simulink model "VCUHVACT"  (R2024b)
settings: Solver=FixedStepDiscrete  StartTime=0.0  StopTime=10.0  FixedStep=0.1  RelTol=1e-3
libraries: simulink x10
settings Model: Creator=32032  LastModifiedBy=32032
settings DataIOCC: SaveFormat=StructureWithTime
settings OptimizationCC: DefaultParameterBehavior=Inlined  UseDivisionForNetSlopeComputation=on  InlineInvariantSignals=on  EnhancedBackFolding=on  PassReuseOutputArgsAs=Individual arguments  ZeroExternalMemoryAtStartup=off  ZeroInternalMemoryAtStartup=off  EfficientFloat2IntCast=on  LifeSpan=inf  OptimizeBlockOrder=speed  DifferentSizesBufferReuse=on  EfficientTunableParamExpr=on
settings DebuggingCC: SignalInfNanChecking=error  ParameterTunabilityLossMsg=error  AssertControl=DisableAll  StrictBusMsg=ErrorOnBusTreatedAsVector
settings ModelReferenceCC: ModelReferenceNumInstancesAllowed=Single
settings SFSimCC: CompileTimeRecursionLimit=0  EnableRuntimeRecursion=off  MATLABDynamicMemAlloc=off
settings RTWCC: Description=AUTOSAR  SystemTargetFile=autosar.tlc  GenCodeOnly=on  TemplateMakefile=ert_default_tmf  DataTypeReplacement=CDataTypesFixedWidth
settings CodeAppCC: ForceParamTrailComments=on  IgnoreCustomStorageClasses=off  IgnoreTestpoints=on  OperatorAnnotations=on  SimulinkDataObjDesc=on  SFDataObjDesc=on  MATLABFcnDesc=on  InsertBlockDesc=on
settings STFCustomTargetCC: TargetLangStandard=C99 (ISO)  UtilityFuncGeneration=Shared location  MultiwordLength=256  ParMdlRefBuildCompliant=on  CompOptLevelCompliant=on  IncludeMdlTerminateFcn=off  CombineOutputUpdateFcns=on  SuppressErrorStatus=on  ERTCustomFileBanners=on  SupportAbsoluteTime=off  SupportNonFinite=off  SupportComplex=off  SupportContinuousTime=off  SupportNonInlinedSFcns=off  RemoveResetFunc=on  ParenthesesLevel=Standards  CastingMode=Standards  MATLABClassNameForMDSCustomization=Simulink.SoftwareTarget.ERTCustomization  AutosarCompliant=on  UseToolchainInfoCompliant=on  GenerateSharedConstants=off  LookupTableObjectStructAxisOrder=2,1,3,4,...  LUTObjectStructOrderEvenSpacing=Size,Table,Breakpoints  SystemTargetFile=autosar.tlc
settings ERTTargetCC: TargetLangStandard=C99 (ISO)  UtilityFuncGeneration=Shared location  ConcurrentExecutionCompliant=off  IncludeMdlTerminateFcn=off  SuppressErrorStatus=on  SupportAbsoluteTime=off  SupportNonFinite=off  SupportComplex=off  ParenthesesLevel=Standards  CastingMode=Standards  ModelStepFunctionPrototypeControlCompliant=off  CPPClassGenCompliant=off  AutosarCompliant=on  GenerateSharedConstants=off  LookupTableObjectStructAxisOrder=2,1,3,4,...  LUTObjectStructOrderEvenSpacing=Size,Table,Breakpoints  ERTCustomFileTemplate=example_file_process.tlc  SuppressUnreachableDefaultCases=off  EnableSignedLeftShifts=off  EnableSignedRightShifts=off  BooleanTrueId=TRUE  BooleanFalseId=FALSE
settings ConfigComp: CovScope=ReferencedModels

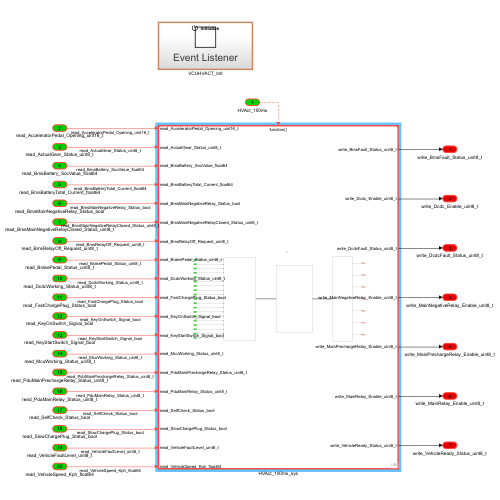
[thumbnail: Simulink's stored preview of the top-level diagram]
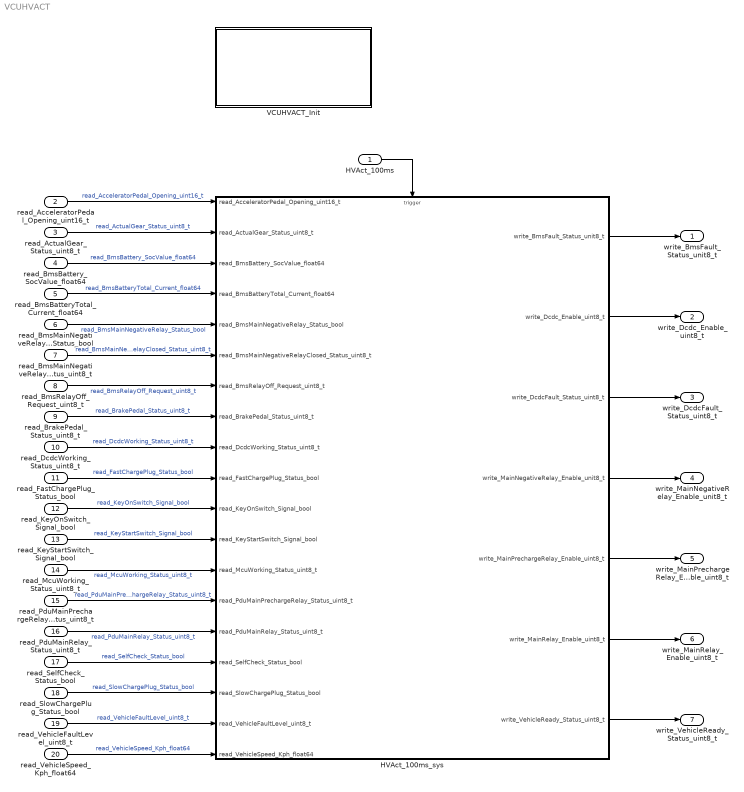
== system VCUHVACT ==
  HVAct_100ms : Inport  SampleTime=0.1  OutputFunctionCall=on
  read_AcceleratorPedal_Opening_uint16_t : Inport  Port=2  OutDataTypeStr=uint16  PortDimensions=1
  read_ActualGear_Status_uint8_t : Inport  Port=3  OutDataTypeStr=uint8  PortDimensions=1
  read_BmsBattery_SocValue_float64 : Inport  Port=4  OutDataTypeStr=double  PortDimensions=1
  read_BmsBatteryTotal_Current_float64 : Inport  Port=5  OutDataTypeStr=double  PortDimensions=1
  read_BmsMainNegativeRelay_Status_bool : Inport  Port=6  OutDataTypeStr=boolean  PortDimensions=1
  read_BmsMainNegativeRelayClosed_Status_uint8_t : Inport  Port=7  OutDataTypeStr=uint8  PortDimensions=1
  read_BmsRelayOff_Request_uint8_t : Inport  Port=8  OutDataTypeStr=uint8  PortDimensions=1
  read_BrakePedal_Status_uint8_t : Inport  Port=9  OutDataTypeStr=uint8  PortDimensions=1
  read_DcdcWorking_Status_uint8_t : Inport  Port=10  OutDataTypeStr=uint8  PortDimensions=1
  read_FastChargePlug_Status_bool : Inport  Port=11  OutDataTypeStr=boolean  PortDimensions=1
  read_KeyOnSwitch_Signal_bool : Inport  Port=12  OutDataTypeStr=boolean  PortDimensions=1
  read_KeyStartSwitch_Signal_bool : Inport  Port=13  OutDataTypeStr=boolean  PortDimensions=1
  read_McuWorking_Status_uint8_t : Inport  Port=14  OutDataTypeStr=uint8  PortDimensions=1
  read_PduMainPrechargeRelay_Status_uint8_t : Inport  Port=15  OutDataTypeStr=uint8  PortDimensions=1
  read_PduMainRelay_Status_uint8_t : Inport  Port=16  OutDataTypeStr=uint8  PortDimensions=1
  read_SelfCheck_Status_bool : Inport  Port=17  OutDataTypeStr=boolean  PortDimensions=1
  read_SlowChargePlug_Status_bool : Inport  Port=18  OutDataTypeStr=boolean  PortDimensions=1
  read_VehicleFaultLevel_uint8_t : Inport  Port=19  OutDataTypeStr=uint8  PortDimensions=1
  read_VehicleSpeed_Kph_float64 : Inport  Port=20  OutDataTypeStr=double  PortDimensions=1
  HVAct_100ms_sys : Subsystem
  VCUHVACT_Init : Subsystem
  write_BmsFault_Status_unit8_t : Outport  OutDataTypeStr=uint8  PortDimensions=1
  write_Dcdc_Enable_uint8_t : Outport  Port=2  OutDataTypeStr=uint8  PortDimensions=1
  write_DcdcFault_Status_uint8_t : Outport  Port=3  OutDataTypeStr=uint8  PortDimensions=1
  write_MainNegativeRelay_Enable_unit8_t : Outport  Port=4  OutDataTypeStr=uint8  PortDimensions=1
  write_MainPrechargeRelay_Enable_uint8_t : Outport  Port=5  OutDataTypeStr=uint8  PortDimensions=1
  write_MainRelay_Enable_uint8_t : Outport  Port=6  OutDataTypeStr=uint8  PortDimensions=1
  write_VehicleReady_Status_uint8_t : Outport  Port=7  OutDataTypeStr=uint8  PortDimensions=1
  wires:
  read_AcceleratorPedal_Opening_uint16_t/1 -> HVAct_100ms_sys/1(read_AcceleratorPedal_Opening_uint16_t)  "read_AcceleratorPedal_Opening_uint16_t"
  read_ActualGear_Status_uint8_t/1 -> HVAct_100ms_sys/2(read_ActualGear_Status_uint8_t)  "read_ActualGear_Status_uint8_t"
  read_BmsBattery_SocValue_float64/1 -> HVAct_100ms_sys/3(read_BmsBattery_SocValue_float64)  "read_BmsBattery_SocValue_float64"
  read_BmsBatteryTotal_Current_float64/1 -> HVAct_100ms_sys/4(read_BmsBatteryTotal_Current_float64)  "read_BmsBatteryTotal_Current_float64"
  read_BmsMainNegativeRelay_Status_bool/1 -> HVAct_100ms_sys/5(read_BmsMainNegativeRelay_Status_bool)  "read_BmsMainNegativeRelay_Status_bool"
  read_BmsMainNegativeRelayClosed_Status_uint8_t/1 -> HVAct_100ms_sys/6(read_BmsMainNegativeRelayClosed_Status_uint8_t)  "read_BmsMainNegativeRelayClosed_Status_uint8_t"
  read_BmsRelayOff_Request_uint8_t/1 -> HVAct_100ms_sys/7(read_BmsRelayOff_Request_uint8_t)  "read_BmsRelayOff_Request_uint8_t"
  read_BrakePedal_Status_uint8_t/1 -> HVAct_100ms_sys/8(read_BrakePedal_Status_uint8_t)  "read_BrakePedal_Status_uint8_t"
  read_DcdcWorking_Status_uint8_t/1 -> HVAct_100ms_sys/9(read_DcdcWorking_Status_uint8_t)  "read_DcdcWorking_Status_uint8_t"
  read_FastChargePlug_Status_bool/1 -> HVAct_100ms_sys/10(read_FastChargePlug_Status_bool)  "read_FastChargePlug_Status_bool"
  read_KeyOnSwitch_Signal_bool/1 -> HVAct_100ms_sys/11(read_KeyOnSwitch_Signal_bool)  "read_KeyOnSwitch_Signal_bool"
  read_KeyStartSwitch_Signal_bool/1 -> HVAct_100ms_sys/12(read_KeyStartSwitch_Signal_bool)  "read_KeyStartSwitch_Signal_bool"
  read_McuWorking_Status_uint8_t/1 -> HVAct_100ms_sys/13(read_McuWorking_Status_uint8_t)  "read_McuWorking_Status_uint8_t"
  read_PduMainPrechargeRelay_Status_uint8_t/1 -> HVAct_100ms_sys/14(read_PduMainPrechargeRelay_Status_uint8_t)  "read_PduMainPrechargeRelay_Status_uint8_t"
  read_PduMainRelay_Status_uint8_t/1 -> HVAct_100ms_sys/15(read_PduMainRelay_Status_uint8_t)  "read_PduMainRelay_Status_uint8_t"
  read_SelfCheck_Status_bool/1 -> HVAct_100ms_sys/16(read_SelfCheck_Status_bool)  "read_SelfCheck_Status_bool"
  read_SlowChargePlug_Status_bool/1 -> HVAct_100ms_sys/17(read_SlowChargePlug_Status_bool)  "read_SlowChargePlug_Status_bool"
  read_VehicleFaultLevel_uint8_t/1 -> HVAct_100ms_sys/18(read_VehicleFaultLevel_uint8_t)  "read_VehicleFaultLevel_uint8_t"
  read_VehicleSpeed_Kph_float64/1 -> HVAct_100ms_sys/19(read_VehicleSpeed_Kph_float64)  "read_VehicleSpeed_Kph_float64"
  HVAct_100ms_sys/1(write_BmsFault_Status_unit8_t) -> write_BmsFault_Status_unit8_t/1
  HVAct_100ms_sys/2(write_Dcdc_Enable_uint8_t) -> write_Dcdc_Enable_uint8_t/1
  HVAct_100ms_sys/3(write_DcdcFault_Status_uint8_t) -> write_DcdcFault_Status_uint8_t/1
  HVAct_100ms_sys/4(write_MainNegativeRelay_Enable_unit8_t) -> write_MainNegativeRelay_Enable_unit8_t/1
  HVAct_100ms_sys/5(write_MainPrechargeRelay_Enable_uint8_t) -> write_MainPrechargeRelay_Enable_uint8_t/1
  HVAct_100ms_sys/6(write_MainRelay_Enable_uint8_t) -> write_MainRelay_Enable_uint8_t/1
  HVAct_100ms_sys/7(write_VehicleReady_Status_uint8_t) -> write_VehicleReady_Status_uint8_t/1
  HVAct_100ms/1 -> HVAct_100ms_sys/Trigger

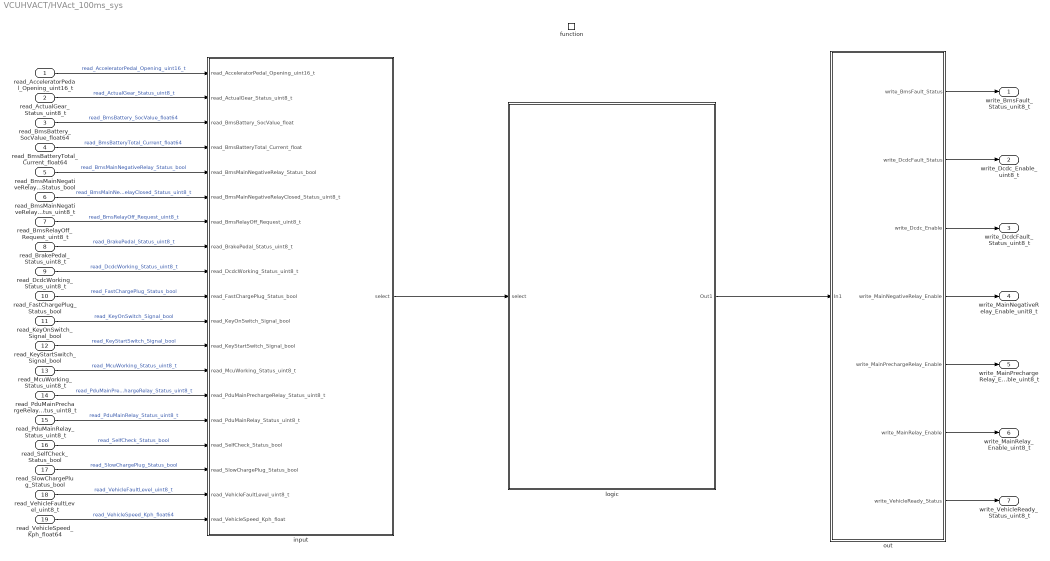
== system VCUHVACT/HVAct_100ms_sys ==
  read_AcceleratorPedal_Opening_uint16_t : Inport
  read_ActualGear_Status_uint8_t : Inport  Port=2
  read_BmsBattery_SocValue_float64 : Inport  Port=3
  read_BmsBatteryTotal_Current_float64 : Inport  Port=4
  read_BmsMainNegativeRelay_Status_bool : Inport  Port=5
  read_BmsMainNegativeRelayClosed_Status_uint8_t : Inport  Port=6
  read_BmsRelayOff_Request_uint8_t : Inport  Port=7
  read_BrakePedal_Status_uint8_t : Inport  Port=8
  read_DcdcWorking_Status_uint8_t : Inport  Port=9
  read_FastChargePlug_Status_bool : Inport  Port=10
  read_KeyOnSwitch_Signal_bool : Inport  Port=11
  read_KeyStartSwitch_Signal_bool : Inport  Port=12
  read_McuWorking_Status_uint8_t : Inport  Port=13
  read_PduMainPrechargeRelay_Status_uint8_t : Inport  Port=14
  read_PduMainRelay_Status_uint8_t : Inport  Port=15
  read_SelfCheck_Status_bool : Inport  Port=16
  read_SlowChargePlug_Status_bool : Inport  Port=17
  read_VehicleFaultLevel_uint8_t : Inport  Port=18
  read_VehicleSpeed_Kph_float64 : Inport  Port=19
  function : TriggerPort  TriggerType=function-call  VariantControl=(inherit)  SampleTimeType=periodic  SampleTime=-1
  input : Subsystem
  logic : Subsystem
  out : Subsystem
  write_BmsFault_Status_unit8_t : Outport
      settings: EnsureOutportIsVirtual=on
  write_Dcdc_Enable_uint8_t : Outport  Port=2
      settings: EnsureOutportIsVirtual=on
  write_DcdcFault_Status_uint8_t : Outport  Port=3
      settings: EnsureOutportIsVirtual=on
  write_MainNegativeRelay_Enable_unit8_t : Outport  Port=4
      settings: EnsureOutportIsVirtual=on
  write_MainPrechargeRelay_Enable_uint8_t : Outport  Port=5
      settings: EnsureOutportIsVirtual=on
  write_MainRelay_Enable_uint8_t : Outport  Port=6
      settings: EnsureOutportIsVirtual=on
  write_VehicleReady_Status_uint8_t : Outport  Port=7
      settings: EnsureOutportIsVirtual=on
  wires:
  read_AcceleratorPedal_Opening_uint16_t/1 -> input/1(read_AcceleratorPedal_Opening_uint16_t)  "read_AcceleratorPedal_Opening_uint16_t"
  read_ActualGear_Status_uint8_t/1 -> input/2(read_ActualGear_Status_uint8_t)  "read_ActualGear_Status_uint8_t"
  read_BmsBattery_SocValue_float64/1 -> input/3(read_BmsBattery_SocValue_float)  "read_BmsBattery_SocValue_float64"
  read_BmsBatteryTotal_Current_float64/1 -> input/4(read_BmsBatteryTotal_Current_float)  "read_BmsBatteryTotal_Current_float64"
  read_BmsMainNegativeRelay_Status_bool/1 -> input/5(read_BmsMainNegativeRelay_Status_bool)  "read_BmsMainNegativeRelay_Status_bool"
  read_BmsMainNegativeRelayClosed_Status_uint8_t/1 -> input/6(read_BmsMainNegativeRelayClosed_Status_uint8_t)  "read_BmsMainNegativeRelayClosed_Status_uint8_t"
  read_BmsRelayOff_Request_uint8_t/1 -> input/7(read_BmsRelayOff_Request_uint8_t)  "read_BmsRelayOff_Request_uint8_t"
  read_BrakePedal_Status_uint8_t/1 -> input/8(read_BrakePedal_Status_uint8_t)  "read_BrakePedal_Status_uint8_t"
  read_DcdcWorking_Status_uint8_t/1 -> input/9(read_DcdcWorking_Status_uint8_t)  "read_DcdcWorking_Status_uint8_t"
  read_FastChargePlug_Status_bool/1 -> input/10(read_FastChargePlug_Status_bool)  "read_FastChargePlug_Status_bool"
  read_KeyOnSwitch_Signal_bool/1 -> input/11(read_KeyOnSwitch_Signal_bool)  "read_KeyOnSwitch_Signal_bool"
  read_KeyStartSwitch_Signal_bool/1 -> input/12(read_KeyStartSwitch_Signal_bool)  "read_KeyStartSwitch_Signal_bool"
  read_McuWorking_Status_uint8_t/1 -> input/13(read_McuWorking_Status_uint8_t)  "read_McuWorking_Status_uint8_t"
  read_PduMainPrechargeRelay_Status_uint8_t/1 -> input/14(read_PduMainPrechargeRelay_Status_uint8_t)  "read_PduMainPrechargeRelay_Status_uint8_t"
  read_PduMainRelay_Status_uint8_t/1 -> input/15(read_PduMainRelay_Status_uint8_t)  "read_PduMainRelay_Status_uint8_t"
  read_SelfCheck_Status_bool/1 -> input/16(read_SelfCheck_Status_bool)  "read_SelfCheck_Status_bool"
  read_SlowChargePlug_Status_bool/1 -> input/17(read_SlowChargePlug_Status_bool)  "read_SlowChargePlug_Status_bool"
  read_VehicleFaultLevel_uint8_t/1 -> input/18(read_VehicleFaultLevel_uint8_t)  "read_VehicleFaultLevel_uint8_t"
  read_VehicleSpeed_Kph_float64/1 -> input/19(read_VehicleSpeed_Kph_float)  "read_VehicleSpeed_Kph_float64"
  input/1(select) -> logic/1(select)
  out/1("write_BmsFault_Status ") -> write_BmsFault_Status_unit8_t/1
  out/2("write_DcdcFault_Status ") -> write_Dcdc_Enable_uint8_t/1
  out/3("write_Dcdc_Enable ") -> write_DcdcFault_Status_uint8_t/1
  out/4("write_MainNegativeRelay_Enable ") -> write_MainNegativeRelay_Enable_unit8_t/1
  out/5("write_MainPrechargeRelay_Enable ") -> write_MainPrechargeRelay_Enable_uint8_t/1
  out/6(write_MainRelay_Enable) -> write_MainRelay_Enable_uint8_t/1
  out/7("write_VehicleReady_Status ") -> write_VehicleReady_Status_uint8_t/1
  logic/1(Out1) -> out/1(In1)

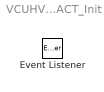
== system VCUHVACT/VCUHVACT_Init ==
  Event Listener : EventListener  EventName=reset

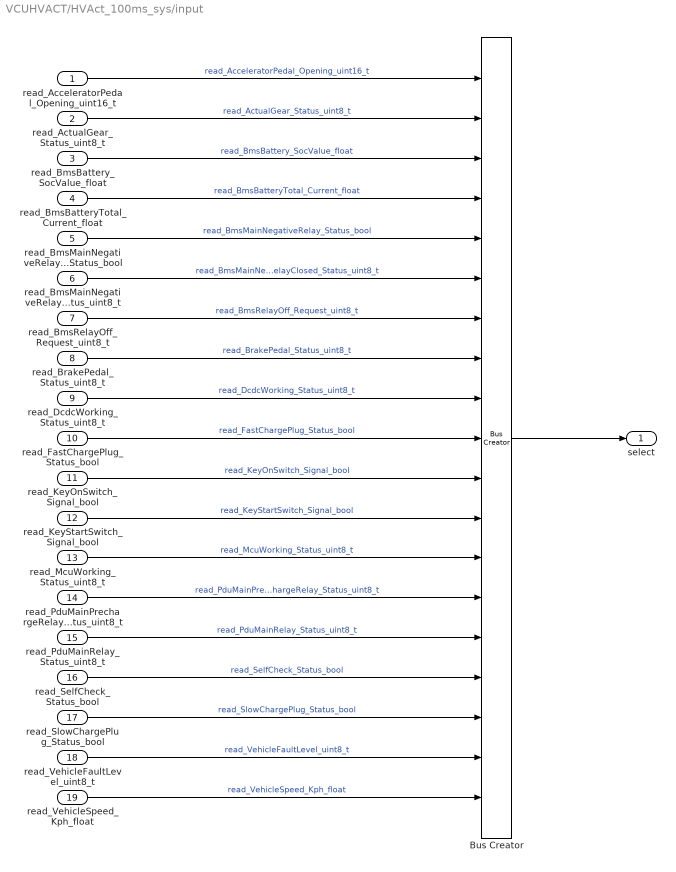
== system VCUHVACT/HVAct_100ms_sys/input ==
  read_AcceleratorPedal_Opening_uint16_t : Inport  OutDataTypeStr=uint16  PortDimensions=1
  read_ActualGear_Status_uint8_t : Inport  Port=2  OutDataTypeStr=uint8  PortDimensions=1
  read_BmsBattery_SocValue_float : Inport  Port=3  OutDataTypeStr=double  PortDimensions=1
  read_BmsBatteryTotal_Current_float : Inport  Port=4  OutDataTypeStr=double  PortDimensions=1
  read_BmsMainNegativeRelay_Status_bool : Inport  Port=5  OutDataTypeStr=boolean  PortDimensions=1
  read_BmsMainNegativeRelayClosed_Status_uint8_t : Inport  Port=6  OutDataTypeStr=uint8  PortDimensions=1
  read_BmsRelayOff_Request_uint8_t : Inport  Port=7  OutDataTypeStr=uint8  PortDimensions=1
  read_BrakePedal_Status_uint8_t : Inport  Port=8  OutDataTypeStr=uint8  PortDimensions=1
  read_DcdcWorking_Status_uint8_t : Inport  Port=9  OutDataTypeStr=uint8  PortDimensions=1
  read_FastChargePlug_Status_bool : Inport  Port=10  OutDataTypeStr=boolean  PortDimensions=1
  read_KeyOnSwitch_Signal_bool : Inport  Port=11  OutDataTypeStr=boolean  PortDimensions=1
  read_KeyStartSwitch_Signal_bool : Inport  Port=12  OutDataTypeStr=boolean  PortDimensions=1
  read_McuWorking_Status_uint8_t : Inport  Port=13  OutDataTypeStr=uint8  PortDimensions=1
  read_PduMainPrechargeRelay_Status_uint8_t : Inport  Port=14  OutDataTypeStr=uint8  PortDimensions=1
  read_PduMainRelay_Status_uint8_t : Inport  Port=15  OutDataTypeStr=uint8  PortDimensions=1
  read_SelfCheck_Status_bool : Inport  Port=16  OutDataTypeStr=boolean  PortDimensions=1
  read_SlowChargePlug_Status_bool : Inport  Port=17  OutDataTypeStr=boolean  PortDimensions=1
  read_VehicleFaultLevel_uint8_t : Inport  Port=18  OutDataTypeStr=uint8  PortDimensions=1
  read_VehicleSpeed_Kph_float : Inport  Port=19  OutDataTypeStr=double  PortDimensions=1
  Bus Creator : BusCreator  Inputs=19
  select : Outport
  wires:
  read_BmsMainNegativeRelayClosed_Status_uint8_t/1 -> Bus Creator/6  "read_BmsMainNegativeRelayClosed_Status_uint8_t"
  read_BmsRelayOff_Request_uint8_t/1 -> Bus Creator/7  "read_BmsRelayOff_Request_uint8_t"
  read_KeyOnSwitch_Signal_bool/1 -> Bus Creator/11  "read_KeyOnSwitch_Signal_bool"
  read_BrakePedal_Status_uint8_t/1 -> Bus Creator/8  "read_BrakePedal_Status_uint8_t"
  read_BmsMainNegativeRelay_Status_bool/1 -> Bus Creator/5  "read_BmsMainNegativeRelay_Status_bool"
  read_BmsBatteryTotal_Current_float/1 -> Bus Creator/4  "read_BmsBatteryTotal_Current_float"
  read_FastChargePlug_Status_bool/1 -> Bus Creator/10  "read_FastChargePlug_Status_bool"
  read_KeyStartSwitch_Signal_bool/1 -> Bus Creator/12  "read_KeyStartSwitch_Signal_bool"
  read_McuWorking_Status_uint8_t/1 -> Bus Creator/13  "read_McuWorking_Status_uint8_t"
  read_SlowChargePlug_Status_bool/1 -> Bus Creator/17  "read_SlowChargePlug_Status_bool"
  read_VehicleFaultLevel_uint8_t/1 -> Bus Creator/18  "read_VehicleFaultLevel_uint8_t"
  read_SelfCheck_Status_bool/1 -> Bus Creator/16  "read_SelfCheck_Status_bool"
  read_PduMainPrechargeRelay_Status_uint8_t/1 -> Bus Creator/14  "read_PduMainPrechargeRelay_Status_uint8_t"
  read_ActualGear_Status_uint8_t/1 -> Bus Creator/2  "read_ActualGear_Status_uint8_t"
  read_AcceleratorPedal_Opening_uint16_t/1 -> Bus Creator/1  "read_AcceleratorPedal_Opening_uint16_t"
  read_VehicleSpeed_Kph_float/1 -> Bus Creator/19  "read_VehicleSpeed_Kph_float"
  read_DcdcWorking_Status_uint8_t/1 -> Bus Creator/9  "read_DcdcWorking_Status_uint8_t"
  read_PduMainRelay_Status_uint8_t/1 -> Bus Creator/15  "read_PduMainRelay_Status_uint8_t"
  read_BmsBattery_SocValue_float/1 -> Bus Creator/3  "read_BmsBattery_SocValue_float"
  Bus Creator/1 -> select/1

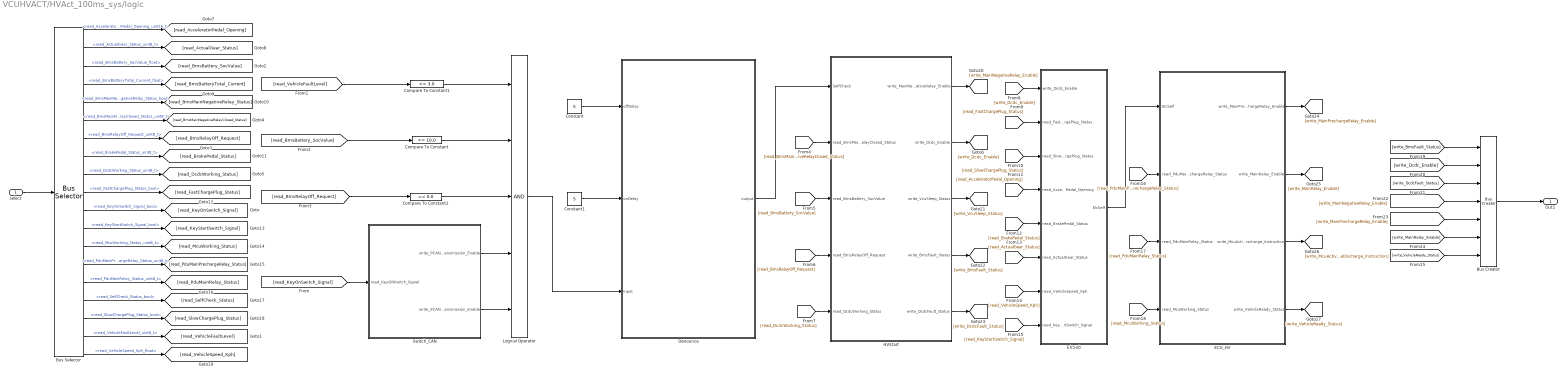
== system VCUHVACT/HVAct_100ms_sys/logic ==
  select : Inport
  Bus Creator : BusCreator  Inputs=7
  Bus Selector : BusSelector  OutputSignals=read_AcceleratorPedal_Opening_uint16_t,read_ActualGear_Status_uint8_t,read_BmsBattery_SocValue_float,read_BmsBatteryTotal_Current_float,read_BmsMainNegativeRelay_Status_bool,read_BmsMainNegativeRelayClosed_Status_uint8_t,read_BmsRelayOff_Request_uint8_t,read_BrakePedal_Status_uint8_t,read_DcdcWorking_Status_uint8_t,read_FastChargePlug_Status_bool,read_KeyOnSwitch_Signal_bool,read_KeyStartSwitch_Signal_bool,read_McuWorking_Status_uint8_t,read_PduMainPrechargeRelay_Status_uint8_t,read_PduMainRelay_Status_uint8_t,read_SelfCheck_Status_bool,read_SlowChargePlug_Status_bool,read_VehicleFaultLevel_uint8_t,read_VehicleSpeed_Kph_float
  Compare To Constant : simulink/Logic and Bit Operations/Compare To Constant  relop=>=  const=10.0  OutDataTypeStr=boolean
  Compare To Constant1 : simulink/Logic and Bit Operations/Compare To Constant  relop=<=  const=3.0  OutDataTypeStr=boolean
  Compare To Constant2 : simulink/Logic and Bit Operations/Compare To Constant  relop===  const=0.0  OutDataTypeStr=boolean
  Constant : Constant  Value=5
  Constant1 : Constant  Value=5
  Denounce : Stateflow chart  TreatAsAtomicUnit=on
  ECU_HV : Stateflow chart  TreatAsAtomicUnit=on
  ElcSub : Subsystem
  HVStart : Stateflow chart  TreatAsAtomicUnit=on
  Logical Operator : Logic  Inputs=5  AllPortsSameDT=off  OutDataTypeStr=boolean
  Switch_CAN : Stateflow chart  TreatAsAtomicUnit=on
  Out1 : Outport
  wires:
  ECU_HV/3(write_McuActiveDischarge_Instruction) -> [write_McuActiveDischarge_Instruction]
  HVStart/2(write_Dcdc_Enable) -> [write_Dcdc_Enable]
  [read_ActualGear_Status] -> ElcSub/6(read_ActualGear_Status)
  Switch_CAN/2(write_ECANTransmission_Enable) -> Logical Operator/5
  [read_BmsBattery_SocValue] -> HVStart/3(read_BmsBattery_SocValue)
  Compare To Constant2/1 -> Logical Operator/3
  [read_BrakePedal_Status] -> ElcSub/5(read_BrakePedal_Status)
  [write_MainRelay_Enable] -> Bus Creator/6
  [read_KeyStartSwitch_Signal] -> ElcSub/8(read_KeyStartSwitch_Signal)
  [read_BmsMainNegativeRelayClosed_Status] -> HVStart/2(read_BmsMainNegativeRelayClosed_Status)
  [write_VehicleReady_Status] -> Bus Creator/7
  Constant1/1 -> Denounce/2(onDelay)
  Denounce/1(output) -> HVStart/1(SelfCheck)
  HVStart/3(write_VcuSleep_Status) -> [write_VcuSleep_Status]
  [read_McuWorking_Status] -> ECU_HV/4(read_McuWorking_Status)
  ECU_HV/4(write_VehicleReady_Status) -> [write_VehicleReady_Status]
  Logical Operator/1 -> Denounce/3(input)
  Constant/1 -> Denounce/1(offDelay)
  [read_KeyOnSwitch_Signal] -> Switch_CAN/1(read_KeyONSwitch_Signal)
  [read_VehicleFaultLevel] -> Compare To Constant1/1
  Compare To Constant/1 -> Logical Operator/2
  ElcSub/1(ElcSelf) -> ECU_HV/1(EIcSelf)
  [read_BmsBattery_SocValue] -> Compare To Constant/1
  HVStart/5(write_DcdcFault_Status) -> [write_DcdcFault_Status]
  [read_SlowChargePlug_Status] -> ElcSub/3(read_SlowChargePlug_Status)
  Compare To Constant1/1 -> Logical Operator/1
  Switch_CAN/1(write_PCANTransmission_Enable) -> Logical Operator/4
  [read_BmsRelayOff_Request] -> HVStart/4(read_BmsRelayOff_Request)
  HVStart/4(write_BmsFault_Status) -> [write_BmsFault_Status]
  [read_BmsRelayOff_Request] -> Compare To Constant2/1
  [read_VehicleSpeed_Kph] -> ElcSub/7(read_VehicleSpeed_Kph)
  [read_DcdcWorking_Status] -> HVStart/5(read_DcdcWorking_Status)
  ECU_HV/1(write_MainPrechargeRelay_Enable) -> [write_MainPrechargeRelay_Enable]
  ECU_HV/2(write_MainRelay_Enable) -> [write_MainRelay_Enable]
  [read_PduMainRelay_Status] -> ECU_HV/3(read_PduMainRelay_Status)
  [write_Dcdc_Enable] -> ElcSub/1(write_Dcdc_Enable)
  [read_AcceleratorPedal_Opening] -> ElcSub/4(read_AcceleratorPedal_Opening)
  [read_PduMainPrechargeRelay_Status] -> ECU_HV/2(read_PduMainPrechargeRelay_Status)
  HVStart/1(write_MainNegativeRelay_Enable) -> [write_MainNegativeRelay_Enable]
  [read_FastChargePlug_Status] -> ElcSub/2(read_FastChargePlug_Status)
  select/1 -> Bus Selector/1
  Bus Selector/1 -> [read_AcceleratorPedal_Opening]  "<read_AcceleratorPedal_Opening_uint16_t>"
  Bus Creator/1 -> Out1/1
  [write_MainPrechargeRelay_Enable] -> Bus Creator/5
  [write_MainNegativeRelay_Enable] -> Bus Creator/4
  [write_DcdcFault_Status] -> Bus Creator/3
  [write_Dcdc_Enable] -> Bus Creator/2
  [write_BmsFault_Status] -> Bus Creator/1
  Bus Selector/19 -> [read_VehicleSpeed_Kph]  "<read_VehicleSpeed_Kph_float>"
  Bus Selector/18 -> [read_VehicleFaultLevel]  "<read_VehicleFaultLevel_uint8_t>"
  Bus Selector/17 -> [read_SlowChargePlug_Status]  "<read_SlowChargePlug_Status_bool>"
  Bus Selector/16 -> [read_SelfCheck_Status]  "<read_SelfCheck_Status_bool>"
  Bus Selector/15 -> [read_PduMainRelay_Status]  "<read_PduMainRelay_Status_uint8_t>"
  Bus Selector/14 -> [read_PduMainPrechargeRelay_Status]  "<read_PduMainPrechargeRelay_Status_uint8_t>"
  Bus Selector/13 -> [read_McuWorking_Status]  "<read_McuWorking_Status_uint8_t>"
  Bus Selector/12 -> [read_KeyStartSwitch_Signal]  "<read_KeyStartSwitch_Signal_bool>"
  Bus Selector/11 -> [read_KeyOnSwitch_Signal]  "<read_KeyOnSwitch_Signal_bool>"
  Bus Selector/10 -> [read_FastChargePlug_Status]  "<read_FastChargePlug_Status_bool>"
  Bus Selector/9 -> [read_DcdcWorking_Status]  "<read_DcdcWorking_Status_uint8_t>"
  Bus Selector/8 -> [read_BrakePedal_Status]  "<read_BrakePedal_Status_uint8_t>"
  Bus Selector/7 -> [read_BmsRelayOff_Request]  "<read_BmsRelayOff_Request_uint8_t>"
  Bus Selector/6 -> [read_BmsMainNegativeRelayClosed_Status]  "<read_BmsMainNegativeRelayClosed_Status_uint8_t>"
  Bus Selector/2 -> [read_ActualGear_Status]  "<read_ActualGear_Status_uint8_t>"
  Bus Selector/3 -> [read_BmsBattery_SocValue]  "<read_BmsBattery_SocValue_float>"
  Bus Selector/4 -> [read_BmsBatteryTotal_Current]  "<read_BmsBatteryTotal_Current_float>"
  Bus Selector/5 -> [read_BmsMainNegativeRelay_Status]  "<read_BmsMainNegativeRelay_Status_bool>"

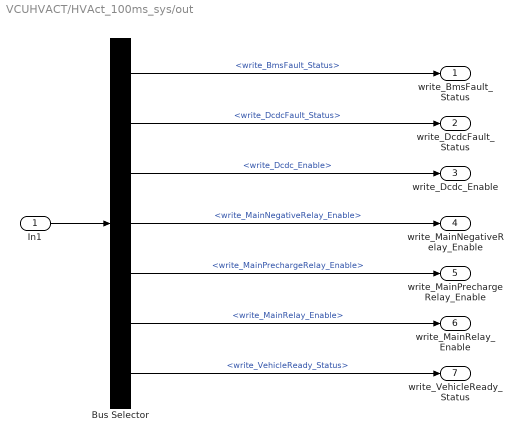
== system VCUHVACT/HVAct_100ms_sys/out ==
  In1 : Inport
  Bus Selector : BusSelector  OutputSignals=write_BmsFault_Status,write_DcdcFault_Status,write_Dcdc_Enable,write_MainNegativeRelay_Enable,write_MainPrechargeRelay_Enable,write_MainRelay_Enable,write_VehicleReady_Status
  "write_BmsFault_Status " : Outport
  "write_DcdcFault_Status " : Outport  Port=2
  "write_Dcdc_Enable " : Outport  Port=3
  "write_MainNegativeRelay_Enable " : Outport  Port=4
  "write_MainPrechargeRelay_Enable " : Outport  Port=5
  write_MainRelay_Enable : Outport  Port=6
  "write_VehicleReady_Status " : Outport  Port=7
  wires:
  In1/1 -> Bus Selector/1
  Bus Selector/2 -> "write_DcdcFault_Status "/1  "<write_DcdcFault_Status>"
  Bus Selector/3 -> "write_Dcdc_Enable "/1  "<write_Dcdc_Enable>"
  Bus Selector/4 -> "write_MainNegativeRelay_Enable "/1  "<write_MainNegativeRelay_Enable>"
  Bus Selector/5 -> "write_MainPrechargeRelay_Enable "/1  "<write_MainPrechargeRelay_Enable>"
  Bus Selector/6 -> write_MainRelay_Enable/1  "<write_MainRelay_Enable>"
  Bus Selector/7 -> "write_VehicleReady_Status "/1  "<write_VehicleReady_Status>"
  Bus Selector/1 -> "write_BmsFault_Status "/1  "<write_BmsFault_Status>"

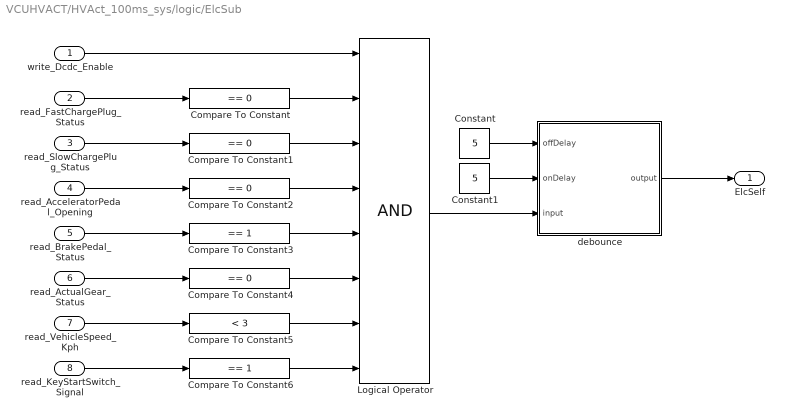
== system VCUHVACT/HVAct_100ms_sys/logic/ElcSub ==
  write_Dcdc_Enable : Inport
  read_FastChargePlug_Status : Inport  Port=2
  read_SlowChargePlug_Status : Inport  Port=3
  read_AcceleratorPedal_Opening : Inport  Port=4
  read_BrakePedal_Status : Inport  Port=5
  read_ActualGear_Status : Inport  Port=6
  read_VehicleSpeed_Kph : Inport  Port=7
  read_KeyStartSwitch_Signal : Inport  Port=8
  Compare To Constant{,1..2,4} (4 alike) : simulink/Logic and Bit Operations/Compare To Constant  relop===  const=0  OutDataTypeStr=boolean
  Compare To Constant3 : simulink/Logic and Bit Operations/Compare To Constant  relop===  const=1  OutDataTypeStr=boolean
  Compare To Constant5 : simulink/Logic and Bit Operations/Compare To Constant  relop=<  const=3  OutDataTypeStr=boolean
  Compare To Constant6 : simulink/Logic and Bit Operations/Compare To Constant  relop===  const=1  OutDataTypeStr=boolean
  Constant : Constant  Value=5
  Constant1 : Constant  Value=5
  Logical Operator : Logic  Inputs=8  AllPortsSameDT=off  OutDataTypeStr=boolean
  debounce : Stateflow chart  TreatAsAtomicUnit=on
  ElcSelf : Outport
  wires:
  read_FastChargePlug_Status/1 -> Compare To Constant/1
  read_SlowChargePlug_Status/1 -> Compare To Constant1/1
  read_AcceleratorPedal_Opening/1 -> Compare To Constant2/1
  read_BrakePedal_Status/1 -> Compare To Constant3/1
  read_ActualGear_Status/1 -> Compare To Constant4/1
  read_VehicleSpeed_Kph/1 -> Compare To Constant5/1
  read_KeyStartSwitch_Signal/1 -> Compare To Constant6/1
  write_Dcdc_Enable/1 -> Logical Operator/1
  Compare To Constant2/1 -> Logical Operator/4
  Compare To Constant3/1 -> Logical Operator/5
  Compare To Constant4/1 -> Logical Operator/6
  Compare To Constant5/1 -> Logical Operator/7
  Compare To Constant6/1 -> Logical Operator/8
  Logical Operator/1 -> debounce/3(input)
  Constant/1 -> debounce/1(offDelay)
  debounce/1(output) -> ElcSelf/1
  Compare To Constant1/1 -> Logical Operator/3
  Compare To Constant/1 -> Logical Operator/2
  Constant1/1 -> debounce/2(onDelay)

== stateflow chart VCUHVACT/HVAct_100ms_sys/logic/ElcSub/debounce ==
  (default) -> (junction 1)
  (junction 6) -> (junction 8) : {counter2 = counter2 + 1;counter1=0;}
  (junction 1) -> (junction 6) [order 1] : [input==0]
  (junction 1) -> (junction 15) [order 2] : [input==1]
  (junction 15) -> (junction 17) : {counter1 = counter1 + 1;counter2==0;}
  (junction 8) -> (junction 12) [order 2]
  (junction 17) -> (junction 12) [order 2]
  (junction 8) -> (junction 10) [order 1] : [counter2>offDelay]
  (junction 17) -> (junction 19) [order 1] : [counter1>onDelay]
  (junction 10) -> (junction 12) : {output=0;counter2=offDelay;}
  (junction 19) -> (junction 12) : {output=1;counter1=onDelay}
  data: offDelay input; onDelay input; output output; counter1 local =0; counter2 local =0; input input

== stateflow chart VCUHVACT/HVAct_100ms_sys/logic/HVStart ==
  state Init
    en:
    write_VcuSleep_Status=0;
    write_MainNegativeRelay_Enable=0;
    write_Dcdc_Enable=0;
    counter=0;
    du:
    counter=counter+1;
  state HV_On
    state HV_ON1
      en:
      write_MainNegativeRelay_Enable=1;
      counter=0;
      du:
      counter=counter+1;
    state HV_ON2
      en:
      counter=0;
      du:
      counter=counter+1;
    state HV_ON3
      en:
      write_Dcdc_Enable=1;
      counter=0;
      du:
      counter=counter+1;
    (default) -> HV_ON1
    HV_ON1 -> HV_ON2 [order 2] : [read_BmsMainNegativeRelayClosed_Status==1]
    HV_ON2 -> HV_ON3 : [counter>=30]
  state HV_OFFStandy
    state HV_OFF2
      en:
      write_MainNegativeRelay_Enable=1;
      counter=0;
      du:
      counter=counter+1;
    state HV_OFF1
      en:
      write_Dcdc_Enable=0;
      counter=0;
      du:
      counter=counter+1;
    HV_OFF1 -> HV_OFF2 : [counter>=30||read_BmsBattery_SocValue<10]
    (default) -> HV_OFF1
  state HV_OFF
    en:
    counter=0;
    du:
    counter=counter+1;
  state HV_Standy
  (default) -> Init
  (junction 36) -> Init
  HV_OFF2 -> (junction 36) [order 2] : [read_BmsRelayOff_Request==1&&SelfCheck~=1]
  (junction 40) -> Init
  HV_OFF2 -> (junction 40) [order 1] : [counter>=30]{write_BmsFault_Status=1}
  Init -> HV_On : [counter>=30&&SelfCheck==1]
  HV_ON1 -> HV_OFF2 [order 1] : [counter>=30]
  HV_On -> HV_OFFStandy : [SelfCheck~=1]
  HV_OFF -> HV_OFFStandy [order 2] : [counter>=30]
  HV_ON3 -> HV_Standy [order 1] : [read_DcdcWorking_Status==1]
  HV_ON3 -> HV_Standy [order 2] : [counter>=30]{write_DcdcFault_Status=1}
  HV_OFF -> HV_Standy [order 1] : [SelfCheck==1]
  HV_Standy -> HV_OFF : [SelfCheck~=1]
  data: counter local; SelfCheck input; write_MainNegativeRelay_Enable output uint8; write_Dcdc_Enable output uint8; write_VcuSleep_Status output uint8; read_BmsMainNegativeRelayClosed_Status input; read_BmsBattery_SocValue input; read_BmsRelayOff_Request input; read_DcdcWorking_Status input; write_BmsFault_Status output uint8; write_DcdcFault_Status output uint8

== stateflow chart VCUHVACT/HVAct_100ms_sys/logic/Switch_CAN ==
  state Init
    write_PCANTransmission_Enable=false;
    write_ECANTransmission_Enable=false;
  state On
    write_PCANTransmission_Enable=true;
    write_ECANTransmission_Enable=true;
  (default) -> Init
  On -> Init : [read_KeyONSwitch_Signal~=1]
  Init -> On : [read_KeyONSwitch_Signal==1]
  data: read_KeyONSwitch_Signal input; write_PCANTransmission_Enable output boolean; write_ECANTransmission_Enable output boolean

== stateflow chart VCUHVACT/HVAct_100ms_sys/logic/Denounce ==
  (default) -> (junction 6)
  (junction 5) -> (junction 1) : {counter2 = counter2 + 1;counter1=0;}
  (junction 6) -> (junction 5) [order 1] : [input==0]
  (junction 6) -> (junction 18) [order 2] : [input==1]
  (junction 18) -> (junction 19) : {counter1 = counter1 + 1;counter2=0;}
  (junction 1) -> (junction 12) [order 2]
  (junction 19) -> (junction 12) [order 2]
  (junction 1) -> (junction 13) [order 1] : [counter2>offDelay]
  (junction 19) -> (junction 11) [order 1] : [counter1>onDelay]
  (junction 13) -> (junction 12) : {output=0;counter2=offDelay;}
  (junction 11) -> (junction 12) : {output=1;counter1=onDelay;}
  data: offDelay input; onDelay input; output output =0; counter1 local =0; counter2 local =0; input input

== stateflow chart VCUHVACT/HVAct_100ms_sys/logic/ECU_HV ==
  state ECU_init
    en:
    write_McuActiveDischarge_Instruction=0;
  state ECU_HVPower
    state ECU_HV1
      en:
      write_MainPrechargeRelay_Enable=1;
      counter=0;
      du:
      counter=counter+1;
    state ECU_HV2
      en:
      write_MainRelay_Enable=1;
      counter=0;
      du:
      counter=counter+1;
    state ECU_HV3
      en:
      counter=0;
      du:
      counter=counter+1;
    state ECU_HV4
      en:
      write_MainPrechargeRelay_Enable=0;
      counter=0;
      du:
      counter=counter+1;
    state ECU_HV5
      en:
      write_VehicleReady_Status=1;
    ECU_HV1 -> ECU_HV2 [order 1] : [read_PduMainPrechargeRelay_Status==1]
    ECU_HV2 -> ECU_HV3 [order 1] : [read_PduMainRelay_Status==1]
    ECU_HV3 -> ECU_HV4 : [counter>=10]
    ECU_HV4 -> ECU_HV5 : [counter>=10]
  state ECU_HVOFF
    state ECU_OFF4
      en:
      write_McuActiveDischarge_Instruction=1;
      counter=0;
      du:
      counter=counter+1;
    state ECU_OFF3
      en:
      counter=0;
      du:
      counter=counter+1;
    state ECU_OFF2
      en:
      write_MainPrechargeRelay_Enable=0;
      write_MainRelay_Enable=0;
    state ECU_OFF1
      en:
      write_VehicleReady_Status=0;
    ECU_OFF3 -> ECU_OFF4 : [counter>=10]
    ECU_OFF2 -> ECU_OFF3 : [read_PduMainRelay_Status==0&&read_PduMainPrechargeRelay_Status==0]
    ECU_OFF1 -> ECU_OFF2
    (default) -> ECU_OFF1
  (default) -> ECU_init
  ECU_init -> ECU_HV1 : [EIcSelf==1]
  ECU_OFF4 -> ECU_init [order 1] : [read_McuWorking_Status==2]
  ECU_OFF4 -> ECU_init [order 2] : [counter>=20]
  ECU_HV1 -> (junction 42) [order 2] : [counter>=30]
  (junction 42) -> (junction 43)
  ECU_HV2 -> (junction 43) [order 2] : [counter>=30]
  (junction 43) -> ECU_OFF2
  ECU_HVPower -> ECU_HVOFF : [EIcSelf==0]
  data: EIcSelf input; read_PduMainPrechargeRelay_Status input; read_PduMainRelay_Status input; write_MainPrechargeRelay_Enable output uint8; counter local; write_MainRelay_Enable output uint8; write_McuActiveDischarge_Instruction output; write_VehicleReady_Status output uint8; read_McuWorking_Status input
